simulink model "LQR"  (R2014a)
settings: Solver=ode3  StartTime=0.0  StopTime=100  FixedStep=0.1  RelTol=1e-3
undefined symbols (not defined in the file or in its folder): alpha
settings Model: Creator=sameer  LastModifiedBy=sameer

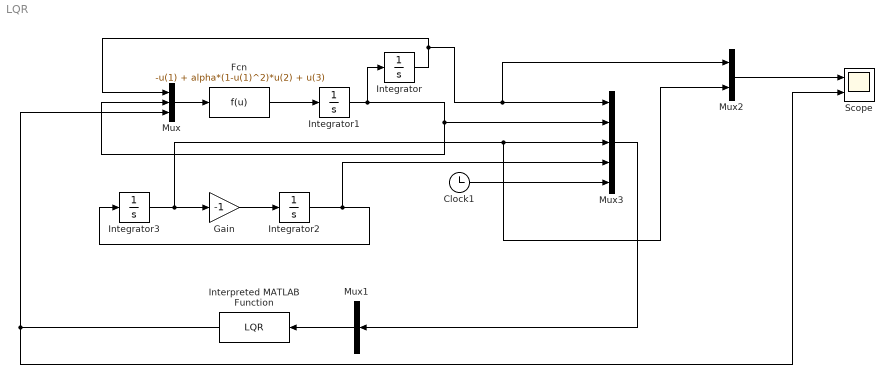
== system LQR ==
  Clock1 : Clock
  Fcn : Fcn  Expr=-u(1) + alpha*(1-u(1)^2)*u(2) + u(3)
  Gain : Gain  Gain=-1
  Integrator : Integrator  InitialCondition=2
  Integrator1 : Integrator  InitialCondition=1
  Integrator2 : Integrator  InitialCondition=1
  Integrator3 : Integrator
  Interpreted MATLAB Function : MATLABFcn  MATLABFcn=LQR
  Mux : Mux  Inputs=3
  Mux1 : Mux  Inputs=1
  Mux2 : Mux  Inputs=2
  Mux3 : Mux  Inputs=5
  Scope : Scope  NumInputPorts=2
      settings: ShowLegends=on  YMin=-5~-5  YMax=5~5
  wires:
  Integrator1/1 -> Mux3/2, Mux/2, Integrator/1
  Mux/1 -> Fcn/1
  Fcn/1 -> Integrator1/1
  Integrator/1 -> Mux/1, Mux2/1, Mux3/1
  Integrator3/1 -> Mux2/2, Mux3/3, Gain/1
  Integrator2/1 -> Mux3/4, Integrator3/1
  Gain/1 -> Integrator2/1
  Mux3/1 -> Mux1/1
  Mux1/1 -> Interpreted MATLAB Function/1
  Mux2/1 -> Scope/1
  Interpreted MATLAB Function/1 -> Scope/2, Mux/3
  Clock1/1 -> Mux3/5
